simulink model "CLIK_pseudoinv_jacob_1order"  (R2021a)
settings: Solver=VariableStepAuto  StartTime=0.0  StopTime=50  RelTol=1e-3
values from neighbouring files (symbols this model uses):
  K = diag([1000 10 100])    [pseudo_traiettoria.m]
  q0 = scara.ikine(T0, 'mask', [1 1 1 1 0 0])    [pseudo_traiettoria.m]    (also in traiettoria.m)
  Tc = 0.001    [pseudo_traiettoria.m]    (also in traiettoria.m)
undefined symbols (not defined in the file or in its folder): DiscIntNeverNeededParam
settings Model: Creator=Ciro  LastModifiedBy=Ciro

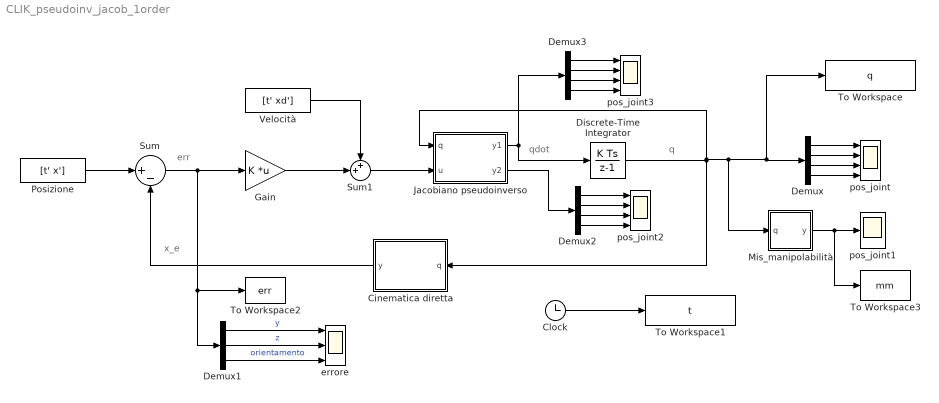
== system CLIK_pseudoinv_jacob_1order ==
  note: err
  note: q
  note: x_e
  note: qdot
  Cinematica diretta : MATLAB Function  TreatAsAtomicUnit=on
  Clock : Clock
  Demux : Demux
  Demux1 : Demux  Outputs=3
  Demux2 : Demux
  Demux3 : Demux
  Discrete-Time Integrator : DiscreteIntegrator  InitialCondition=q0  SampleTime=Tc  ICPrevOutput=DiscIntNeverNeededParam  ICPrevScaledInput=DiscIntNeverNeededParam
  Gain : Gain  Gain=K  Multiplication=Matrix(K*u)
  Jacobiano pseudoinverso : MATLAB Function  TreatAsAtomicUnit=on
  Mis_manipolabilità : MATLAB Function  TreatAsAtomicUnit=on
  Posizione : FromWorkspace  VariableName=[t' x']  OutDataTypeStr=double  SampleTime=Tc  OutputAfterFinalValue=Holding final value
  Sum : Sum  Inputs=|+-
  Sum1 : Sum  Inputs=++|
  To Workspace : ToWorkspace  VariableName=q  SampleTime=Tc
      settings: Save2DSignal=2-D array (concatenate along first dimension)
  To Workspace1 : ToWorkspace  VariableName=t  SampleTime=Tc
      settings: Save2DSignal=2-D array (concatenate along first dimension)
  To Workspace2 : ToWorkspace  VariableName=err  SampleTime=Tc
      settings: Save2DSignal=2-D array (concatenate along first dimension)
  To Workspace3 : ToWorkspace  VariableName=mm  SampleTime=Tc
      settings: Save2DSignal=2-D array (concatenate along first dimension)
  Velocità : FromWorkspace  VariableName=[t' xd']  OutDataTypeStr=double  SampleTime=Tc  OutputAfterFinalValue=Holding final value
  errore : Scope  NumInputPorts=3
  pos_joint : Scope  NumInputPorts=4
  pos_joint1 : Scope
  pos_joint2 : Scope  NumInputPorts=4
  pos_joint3 : Scope  NumInputPorts=4
  wires:
  Discrete-Time Integrator/1 -> Jacobiano pseudoinverso/1(q), Mis_manipolabilità/1(q), To Workspace/1, Demux/1, Cinematica diretta/1(q)
  Demux/2 -> pos_joint/2
  Sum/1 -> To Workspace2/1, Demux1/1, Gain/1
  Demux/1 -> pos_joint/1
  Cinematica diretta/1(y) -> Sum/2
  Demux/3 -> pos_joint/3
  Demux/4 -> pos_joint/4
  Posizione/1 -> Sum/1
  Sum1/1 -> Jacobiano pseudoinverso/2(u)
  Gain/1 -> Sum1/2
  Velocità/1 -> Sum1/1
  Demux1/3 -> errore/3  "orientamento"
  Demux1/1 -> errore/1  "y"
  Demux1/2 -> errore/2  "z"
  Clock/1 -> To Workspace1/1
  Mis_manipolabilità/1(y) -> To Workspace3/1, pos_joint1/1
  Demux2/4 -> pos_joint2/4
  Demux2/3 -> pos_joint2/3
  Demux2/1 -> pos_joint2/1
  Demux2/2 -> pos_joint2/2
  Jacobiano pseudoinverso/2(y2) -> Demux2/1
  Demux3/4 -> pos_joint3/4
  Demux3/3 -> pos_joint3/3
  Demux3/1 -> pos_joint3/1
  Demux3/2 -> pos_joint3/2
  Jacobiano pseudoinverso/1(y1) -> Demux3/1, Discrete-Time Integrator/1

== matlab function CLIK_pseudoinv_jacob_1order/Jacobiano pseudoinverso ==
  data: q input; u input; y1 output; y2 output
function [y1,y2] = fcn(q, u)

J = [  %-0.5*(sin(q(1))+sin(q(1)+q(2)))  -0.5*sin(q(1)+q(2))  0  0;
     0.5*(cos(q(1))+cos(q(1)+q(2)))  0.5*cos(q(1)+q(2))  0  0;
     0                               0                  -1  0;
     1                               1                   0 -1];
  
Jdag = (J')*inv(J*J');
theta1 = q(1);
theta2 = q(2);
k0=1;
grad_w = [-(cos(theta1)*sin(theta1) + cos(theta1 + theta2)*sin(theta1 + theta2) + (cos(theta1 + theta2)*sin(theta1))/2 + (sin(theta1 + theta2)*cos(theta1))/2)/(2*(cos(theta1 + theta2)^2/2 + cos(theta1)^2/2 + (cos(theta1 + theta2)*cos(theta1))/2)^(1/2));
           -(cos(theta1 + theta2)*sin(theta1 + theta2) + (sin(theta1 + theta2)*cos(theta1))/2)/(2*(cos(theta1 + theta2)^2/2 + cos(theta1)^2/2 + (cos(theta1 + theta2)*cos(theta1))/2)^(1/2));
            0;
            0];
    %w=sqrt(det(J*J'));
%     den = 1/(sqrt(cos(q(1)+q(2))*cos(q(1)+q(2)) + cos(q(1))*cos(q(1)) + cos(q(1))*cos(q(1)+q(2))));
%     grad_w = -(sqrt(2)/4)*[2*cos(q(1)+q(2))*sin(q(1)+q(2)) + 2*cos(q(1))*sin(q(1)) + sin(2*q(1)+q(2));
%         2*cos(q(1)+q(2))*sin(q(1)+q(2)) + cos(q(1))*sin(q(1)+q(2));
%         0;
%         0]*den;

%     den = 1/(sqrt(sin(q(1)+q(2))*sin(q(1)+q(2)) + sin(q(1))*sin(q(1)) + sin(q(1))*sin(q(1)+q(2))));
%     grad_w = (sqrt(2)/4)*[2*sin(q(1)+q(2))*cos(q(1)+q(2)) + 2*sin(q(1))*cos(q(1)) + sin(2*q(1)+q(2));
%         2*sin(q(1)+q(2))*cos(q(1)+q(2)) + sin(q(1))*cos(q(1)+q(2));
%         0;
%         0]*den;

qdot0=k0*grad_w;
y1 = Jdag*u+(eye(4)-Jdag*J)*qdot0;
%
y2 = (eye(4)-Jdag*J)*qdot0;

== matlab function CLIK_pseudoinv_jacob_1order/Mis_manipolabilità ==
  data: q input; y output
function y = fcn(q)

theta1 = q(1);
theta2 = q(2);
mm = sqrt(0.5*cos(theta1 + theta2)^2 + 0.5*cos(theta1)^2 + 0.5*cos(theta1 + theta2)*cos(theta1));
y = mm;

== matlab function CLIK_pseudoinv_jacob_1order/Cinematica diretta ==
  data: q input; y output
function y = fcn(q)

xe = [%0.5*(cos(q(1))+cos(q(1)+q(2)));
      0.5*(sin(q(1))+sin(q(1)+q(2)));
      0.8-q(3);
      q(1)+q(2)-q(4)];

y = xe;
